simulink model "gbell_mf1"  (R2016a)
settings: Solver=ode45  StartTime=0.0  StopTime=10.0  RelTol=1e-3
undefined symbols (not defined in the file): fi_1_a, fi_1_b, fi_1_c
settings Model: Creator=Руслан  LastModifiedBy=Руслан
settings DataIOCC: LimitDataPoints=on  SaveFormat=Array
settings DebuggingCC: AlgebraicLoopMsg=error
settings HardwareCC: ProdBitPerLong=64  ProdLargestAtomicFloat=None  ProdHWDeviceType=Intel->x86-64
settings ModelReferenceCC: PropagateSignalLabelsOutOfModel=off
settings RTWCC: TemplateMakefile=RTW.MSVCBuild  Description=Create Visual C/C++ Solution File for Simulink Coder  GenerateReport=on  RetainRTWFile=on  LaunchReport=on
settings CodeAppCC: ForceParamTrailComments=on  MATLABSourceComments=on
settings GRTTargetCC: TargetLangStandard=C99 (ISO)
settings ConfigComp: CovModelRefEnable=Off

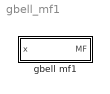
== system gbell_mf1 ==
  gbell mf1 : Subsystem  mask{a=fi_1_a, b=fi_1_b, c=fi_1_c}

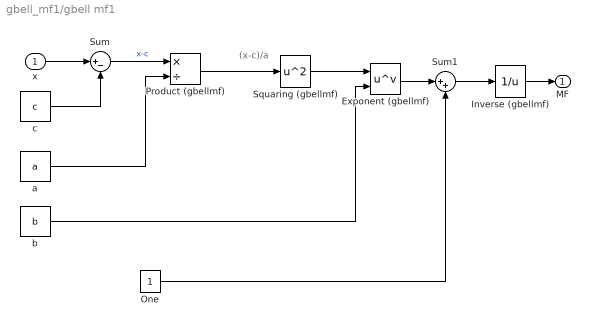
== system gbell_mf1/gbell mf1 ==
  note: (x-c)/a
  x : Inport
  Exponent (gbellmf) : Math  Operator=pow  SaturateOnIntegerOverflow=on
  Inverse (gbellmf) : Math  Operator=reciprocal  SaturateOnIntegerOverflow=on
  One : Constant
  Product (gbellmf) : Product  Inputs=*/  SaturateOnIntegerOverflow=on  InputSameDT=on  OutDataTypeStr=Inherit: Same as first input
  Squaring (gbellmf) : Math  Operator=square  SaturateOnIntegerOverflow=on
  Sum : Sum  Inputs=|+-  SaturateOnIntegerOverflow=on  InputSameDT=on  OutDataTypeStr=Inherit: Same as first input
  Sum1 : Sum  Inputs=|++  SaturateOnIntegerOverflow=on  InputSameDT=on  OutDataTypeStr=Inherit: Same as first input
  a : Constant  Value=a
  b : Constant  Value=b
  c : Constant  Value=c
  MF : Outport
  wires:
  Inverse (gbellmf)/1 -> MF/1
  Sum1/1 -> Inverse (gbellmf)/1
  One/1 -> Sum1/2
  Exponent (gbellmf)/1 -> Sum1/1
  x/1 -> Sum/1
  c/1 -> Sum/2
  Sum/1 -> Product (gbellmf)/1  "x-c"
  a/1 -> Product (gbellmf)/2
  Product (gbellmf)/1 -> Squaring (gbellmf)/1
  Squaring (gbellmf)/1 -> Exponent (gbellmf)/1
  b/1 -> Exponent (gbellmf)/2
